simulink model "FinalProjectSimulinkModel_STAIRS"  (R2023b)
settings: Solver=VariableStepAuto  StartTime=0.0  StopTime=5  RelTol=1e-3
values from neighbouring files (symbols this model uses):
  dq_d_COM = [0.75; 0; 0; 0; 0; 0]    [FinalProject_init.m]
  dtMPC = 0.03    [FinalProject_init.m]
  firstStairDist = 0.26    [FinalProject_init.m]
  kd_swing = 10    [FinalProject_init.m]
  kp_swing = 300    [FinalProject_init.m]
  kStep = 0.001    [FinalProject_init.m]
  NMPC = 10    [FinalProject_init.m]
  offsets = [0;tSwing;tSwing;0]    [FinalProject_init.m]
  q_hip_roll_i = 0    [FinalProject_init.m]
  Qmpc = diag([100 100 50 1000 1000 500 4 4 4 1 1 1 0])    [FinalProject_init.m]
  Rmpc = 0.00001*eye(12)    [FinalProject_init.m]
  task = 6    [FinalProject_init.m]
  tCycle = 0.3    [FinalProject_init.m]
  tRamp = 0.5    [FinalProject_init.m]
  tSwing = tCycle/2    (= 0.15)    [FinalProject_init.m]
  x0_Trunk = [0;0;z_trunk_i-.15; 0;-0.271;0]    [FinalProject_init.m]
undefined symbols (not defined in the file or in its folder): X, Y, Z
libraries: sm_lib x208, nesl_utility x53
(part 5 of 5)

== system FinalProjectSimulinkModel_STAIRS/Rear Right Leg/Rear Right Thigh/RR_thigh ==
  Inertia : sm_lib/Body Elements/Inertia  InertiaType=Custom  Mass=1.013  MassUnits=kg  CenterOfMass=[0, 0, 0]  CenterOfMassUnits=m  MomentsOfInertia=[0.005529065, 0.005139339, 0.001367788]  MomentsOfInertiaUnits=kg*m^2  ProductsOfInertia=[-2.2448e-05, 0.000343869, -4.825e-06]  ProductsOfInertiaUnits=kg*m^2  GraphicType=None  MarkerShape=Inertia  MarkerSize=20  GraphicVisPropType=SimpleVisualProperties  GraphicDiffuseColor=[0.5 0.5 0.5]  GraphicSpecularColor=[0.5 0.5 0.5 1.0]  GraphicAmbientColor=[0.15 0.15 0.15 1.0]  GraphicEmissiveColor=[0.0 0.0 0.0 1.0]  GraphicShininess=75  GraphicOpacity=1.0
  InertiaOriginTransform : sm_lib/Frames and Transforms/Rigid Transform  TranslationMethod=Cartesian  TranslationStandardOffset=0  TranslationStandardOffsetUnits=m  TranslationStandardAxis=+Z  TranslationCartesianOffset=[-0.003237, 0.022327, -0.027326]  TranslationCartesianOffsetUnits=m  TranslationROffset=0  TranslationROffsetUnits=m  TranslationZOffset=0  TranslationZOffsetUnits=m  TranslationThetaOffset=0  TranslationThetaOffsetUnits=deg  RotationMethod=RotationSequence  RotationAngleUnits=deg  RotationStandardAxis=+Z  RotationAngle=0.0  RotationArbitraryAxis=[0 0 1]  FollAlignAxisA=+X  BaseAlignAxisA=+Y  FollAlignAxisB=+Y  BaseAlignAxisB=+Z  RotationSequenceAxes=BaseAxes  RotationSequence=XYZ  RotationSequenceAngles=[0, 0, 0]  RotationSequenceAnglesUnits=rad  RotationMatrix=[1 0 0; 0 1 0; 0 0 1]  Quaternion=[1 0 0 0]
  RR_calf_joint_AxisTransform : sm_lib/Frames and Transforms/Rigid Transform  TranslationMethod=Cartesian  TranslationStandardOffset=0  TranslationStandardOffsetUnits=m  TranslationStandardAxis=+Z  TranslationCartesianOffset=[0, 0, 0]  TranslationCartesianOffsetUnits=m  TranslationROffset=0  TranslationROffsetUnits=m  TranslationZOffset=0  TranslationZOffsetUnits=m  TranslationThetaOffset=0  TranslationThetaOffsetUnits=deg  RotationMethod=ArbitraryAxis  RotationAngleUnits=rad  RotationStandardAxis=+Z  RotationAngle=1.570796326794897  RotationArbitraryAxis=[-1, 0, 0]  FollAlignAxisA=+X  BaseAlignAxisA=+Y  FollAlignAxisB=+Y  BaseAlignAxisB=+Z  RotationSequenceAxes=FollowerAxes  RotationSequence=XYX  RotationSequenceAngles=[0 0 0]  RotationSequenceAnglesUnits=deg  RotationMatrix=[1 0 0; 0 1 0; 0 0 1]  Quaternion=[1 0 0 0]
  RR_calf_joint_OriginTransform : sm_lib/Frames and Transforms/Rigid Transform  TranslationMethod=Cartesian  TranslationStandardOffset=0  TranslationStandardOffsetUnits=m  TranslationStandardAxis=+Z  TranslationCartesianOffset=[0, 0, -0.2]  TranslationCartesianOffsetUnits=m  TranslationROffset=0  TranslationROffsetUnits=m  TranslationZOffset=0  TranslationZOffsetUnits=m  TranslationThetaOffset=0  TranslationThetaOffsetUnits=deg  RotationMethod=RotationSequence  RotationAngleUnits=deg  RotationStandardAxis=+Z  RotationAngle=0.0  RotationArbitraryAxis=[0 0 1]  FollAlignAxisA=+X  BaseAlignAxisA=+Y  FollAlignAxisB=+Y  BaseAlignAxisB=+Z  RotationSequenceAxes=BaseAxes  RotationSequence=XYZ  RotationSequenceAngles=[0, 0, 0]  RotationSequenceAnglesUnits=rad  RotationMatrix=[1 0 0; 0 1 0; 0 0 1]  Quaternion=[1 0 0 0]
  RR_thigh_joint_AxisInvTransform : sm_lib/Frames and Transforms/Rigid Transform  TranslationMethod=Cartesian  TranslationStandardOffset=0  TranslationStandardOffsetUnits=m  TranslationStandardAxis=+Z  TranslationCartesianOffset=[0, 0, 0]  TranslationCartesianOffsetUnits=m  TranslationROffset=0  TranslationROffsetUnits=m  TranslationZOffset=0  TranslationZOffsetUnits=m  TranslationThetaOffset=0  TranslationThetaOffsetUnits=deg  RotationMethod=ArbitraryAxis  RotationAngleUnits=rad  RotationStandardAxis=+Z  RotationAngle=1.570796326794897  RotationArbitraryAxis=[-1, 0, 0]  FollAlignAxisA=+X  BaseAlignAxisA=+Y  FollAlignAxisB=+Y  BaseAlignAxisB=+Z  RotationSequenceAxes=FollowerAxes  RotationSequence=XYX  RotationSequenceAngles=[0 0 0]  RotationSequenceAnglesUnits=deg  RotationMatrix=[1 0 0; 0 1 0; 0 0 1]  Quaternion=[1 0 0 0]
  ReferenceFrame : sm_lib/Frames and Transforms/Reference Frame
  Visual : sm_lib/Body Elements/File Solid  ExtGeomFileName=a1_description/meshes/thigh_mirror.stl  UnitType=Custom  ExtGeomFileUnits=m  StepReaderType=HEX  ExportConvexHullGeometry=off  InertiaType=Custom  Mass=0  MassUnits=kg  CenterOfMass=[0, 0, 0]  CenterOfMassUnits=m  MomentsOfInertia=[0, 0, 0]  MomentsOfInertiaUnits=kg*m^2  ProductsOfInertia=[0, 0, 0]  ProductsOfInertiaUnits=kg*m^2  BasedOnType=DensityFromFile  Density=1000  DensityUnits=kg/m^3  DoExposeReferenceFrame=on  SerializedFrames=<Frames/>  GraphicType=FromGeometry  MarkerShape=Sphere  MarkerSize=10  GraphicVisPropType=SimpleVisualProperties  GraphicDiffuseColor=[0.6 0.6 0.6]  GraphicSpecularColor=[0.5 0.5 0.5 1.0]  GraphicAmbientColor=[0.15 0.15 0.15 1.0]  GraphicEmissiveColor=[0.0 0.0 0.0 1.0]  GraphicShininess=75  GraphicOpacity=1
  VisualOriginTransform : sm_lib/Frames and Transforms/Rigid Transform  TranslationMethod=Cartesian  TranslationStandardOffset=0  TranslationStandardOffsetUnits=m  TranslationStandardAxis=+Z  TranslationCartesianOffset=[0, 0, 0]  TranslationCartesianOffsetUnits=m  TranslationROffset=0  TranslationROffsetUnits=m  TranslationZOffset=0  TranslationZOffsetUnits=m  TranslationThetaOffset=0  TranslationThetaOffsetUnits=deg  RotationMethod=RotationSequence  RotationAngleUnits=deg  RotationStandardAxis=+Z  RotationAngle=0.0  RotationArbitraryAxis=[0 0 1]  FollAlignAxisA=+X  BaseAlignAxisA=+Y  FollAlignAxisB=+Y  BaseAlignAxisB=+Z  RotationSequenceAxes=BaseAxes  RotationSequence=XYZ  RotationSequenceAngles=[0, 0, 0]  RotationSequenceAnglesUnits=rad  RotationMatrix=[1 0 0; 0 1 0; 0 0 1]  Quaternion=[1 0 0 0]
  F : PMIOPort  Side=Left
  F1 : PMIOPort  Port=2  Side=Right
  connections:
  Inertia/RConn1 -- InertiaOriginTransform/RConn1
  RR_calf_joint_AxisTransform/RConn1 -- F1/RConn1
  RR_calf_joint_AxisTransform/LConn1 -- RR_calf_joint_OriginTransform/RConn1
  RR_thigh_joint_AxisInvTransform/RConn1 -- F/RConn1
  RR_calf_joint_OriginTransform/LConn1 -- InertiaOriginTransform/LConn1 -- ReferenceFrame/RConn1 -- VisualOriginTransform/LConn1 -- RR_thigh_joint_AxisInvTransform/LConn1
  Visual/RConn1 -- VisualOriginTransform/RConn1

== system FinalProjectSimulinkModel_STAIRS/Rear Right Leg/Rear Right Calf and Foot/RR_calf ==
  Inertia : sm_lib/Body Elements/Inertia  InertiaType=Custom  Mass=0.166  MassUnits=kg  CenterOfMass=[0, 0, 0]  CenterOfMassUnits=m  MomentsOfInertia=[0.002997972, 0.003014022, 3.2426e-05]  MomentsOfInertiaUnits=kg*m^2  ProductsOfInertia=[0, -0.000141163, 0]  ProductsOfInertiaUnits=kg*m^2  GraphicType=None  MarkerShape=Inertia  MarkerSize=20  GraphicVisPropType=SimpleVisualProperties  GraphicDiffuseColor=[0.5 0.5 0.5]  GraphicSpecularColor=[0.5 0.5 0.5 1.0]  GraphicAmbientColor=[0.15 0.15 0.15 1.0]  GraphicEmissiveColor=[0.0 0.0 0.0 1.0]  GraphicShininess=75  GraphicOpacity=1.0
  InertiaOriginTransform : sm_lib/Frames and Transforms/Rigid Transform  TranslationMethod=Cartesian  TranslationStandardOffset=0  TranslationStandardOffsetUnits=m  TranslationStandardAxis=+Z  TranslationCartesianOffset=[0.006435, 0, -0.107388]  TranslationCartesianOffsetUnits=m  TranslationROffset=0  TranslationROffsetUnits=m  TranslationZOffset=0  TranslationZOffsetUnits=m  TranslationThetaOffset=0  TranslationThetaOffsetUnits=deg  RotationMethod=RotationSequence  RotationAngleUnits=deg  RotationStandardAxis=+Z  RotationAngle=0.0  RotationArbitraryAxis=[0 0 1]  FollAlignAxisA=+X  BaseAlignAxisA=+Y  FollAlignAxisB=+Y  BaseAlignAxisB=+Z  RotationSequenceAxes=BaseAxes  RotationSequence=XYZ  RotationSequenceAngles=[0, 0, 0]  RotationSequenceAnglesUnits=rad  RotationMatrix=[1 0 0; 0 1 0; 0 0 1]  Quaternion=[1 0 0 0]
  RR_calf_joint_AxisInvTransform : sm_lib/Frames and Transforms/Rigid Transform  TranslationMethod=Cartesian  TranslationStandardOffset=0  TranslationStandardOffsetUnits=m  TranslationStandardAxis=+Z  TranslationCartesianOffset=[0, 0, 0]  TranslationCartesianOffsetUnits=m  TranslationROffset=0  TranslationROffsetUnits=m  TranslationZOffset=0  TranslationZOffsetUnits=m  TranslationThetaOffset=0  TranslationThetaOffsetUnits=deg  RotationMethod=ArbitraryAxis  RotationAngleUnits=rad  RotationStandardAxis=+Z  RotationAngle=1.570796326794897  RotationArbitraryAxis=[-1, 0, 0]  FollAlignAxisA=+X  BaseAlignAxisA=+Y  FollAlignAxisB=+Y  BaseAlignAxisB=+Z  RotationSequenceAxes=FollowerAxes  RotationSequence=XYX  RotationSequenceAngles=[0 0 0]  RotationSequenceAnglesUnits=deg  RotationMatrix=[1 0 0; 0 1 0; 0 0 1]  Quaternion=[1 0 0 0]
  RR_foot_fixed_OriginTransform : sm_lib/Frames and Transforms/Rigid Transform  TranslationMethod=Cartesian  TranslationStandardOffset=0  TranslationStandardOffsetUnits=m  TranslationStandardAxis=+Z  TranslationCartesianOffset=[0, 0, -0.2]  TranslationCartesianOffsetUnits=m  TranslationROffset=0  TranslationROffsetUnits=m  TranslationZOffset=0  TranslationZOffsetUnits=m  TranslationThetaOffset=0  TranslationThetaOffsetUnits=deg  RotationMethod=RotationSequence  RotationAngleUnits=deg  RotationStandardAxis=+Z  RotationAngle=0.0  RotationArbitraryAxis=[0 0 1]  FollAlignAxisA=+X  BaseAlignAxisA=+Y  FollAlignAxisB=+Y  BaseAlignAxisB=+Z  RotationSequenceAxes=BaseAxes  RotationSequence=XYZ  RotationSequenceAngles=[0, 0, 0]  RotationSequenceAnglesUnits=rad  RotationMatrix=[1 0 0; 0 1 0; 0 0 1]  Quaternion=[1 0 0 0]
  ReferenceFrame : sm_lib/Frames and Transforms/Reference Frame
  Visual : sm_lib/Body Elements/File Solid  ExtGeomFileName=a1_description/meshes/calf.stl  UnitType=Custom  ExtGeomFileUnits=m  StepReaderType=HEX  ExportConvexHullGeometry=off  InertiaType=Custom  Mass=0  MassUnits=kg  CenterOfMass=[0, 0, 0]  CenterOfMassUnits=m  MomentsOfInertia=[0, 0, 0]  MomentsOfInertiaUnits=kg*m^2  ProductsOfInertia=[0, 0, 0]  ProductsOfInertiaUnits=kg*m^2  BasedOnType=DensityFromFile  Density=1000  DensityUnits=kg/m^3  DoExposeReferenceFrame=on  SerializedFrames=<Frames/>  GraphicType=FromGeometry  MarkerShape=Sphere  MarkerSize=10  GraphicVisPropType=SimpleVisualProperties  GraphicDiffuseColor=[0.2 0.2 0.2]  GraphicSpecularColor=[0.5 0.5 0.5 1.0]  GraphicAmbientColor=[0.15 0.15 0.15 1.0]  GraphicEmissiveColor=[0.0 0.0 0.0 1.0]  GraphicShininess=75  GraphicOpacity=1
  VisualOriginTransform : sm_lib/Frames and Transforms/Rigid Transform  TranslationMethod=Cartesian  TranslationStandardOffset=0  TranslationStandardOffsetUnits=m  TranslationStandardAxis=+Z  TranslationCartesianOffset=[0, 0, 0]  TranslationCartesianOffsetUnits=m  TranslationROffset=0  TranslationROffsetUnits=m  TranslationZOffset=0  TranslationZOffsetUnits=m  TranslationThetaOffset=0  TranslationThetaOffsetUnits=deg  RotationMethod=RotationSequence  RotationAngleUnits=deg  RotationStandardAxis=+Z  RotationAngle=0.0  RotationArbitraryAxis=[0 0 1]  FollAlignAxisA=+X  BaseAlignAxisA=+Y  FollAlignAxisB=+Y  BaseAlignAxisB=+Z  RotationSequenceAxes=BaseAxes  RotationSequence=XYZ  RotationSequenceAngles=[0, 0, 0]  RotationSequenceAnglesUnits=rad  RotationMatrix=[1 0 0; 0 1 0; 0 0 1]  Quaternion=[1 0 0 0]
  F : PMIOPort  Side=Left
  F1 : PMIOPort  Port=2  Side=Right
  connections:
  Inertia/RConn1 -- InertiaOriginTransform/RConn1
  RR_calf_joint_AxisInvTransform/RConn1 -- F/RConn1
  RR_foot_fixed_OriginTransform/RConn1 -- F1/RConn1
  RR_calf_joint_AxisInvTransform/LConn1 -- InertiaOriginTransform/LConn1 -- ReferenceFrame/RConn1 -- VisualOriginTransform/LConn1 -- RR_foot_fixed_OriginTransform/LConn1
  Visual/RConn1 -- VisualOriginTransform/RConn1

== system FinalProjectSimulinkModel_STAIRS/Rear Right Leg/Rear Right Calf and Foot/RR_foot ==
  Inertia : sm_lib/Body Elements/Inertia  InertiaType=Custom  Mass=0.06  MassUnits=kg  CenterOfMass=[0, 0, 0]  CenterOfMassUnits=m  MomentsOfInertia=[9.6e-06, 9.6e-06, 9.6e-06]  MomentsOfInertiaUnits=kg*m^2  ProductsOfInertia=[0, 0, 0]  ProductsOfInertiaUnits=kg*m^2  GraphicType=None  MarkerShape=Inertia  MarkerSize=20  GraphicVisPropType=SimpleVisualProperties  GraphicDiffuseColor=[0.5 0.5 0.5]  GraphicSpecularColor=[0.5 0.5 0.5 1.0]  GraphicAmbientColor=[0.15 0.15 0.15 1.0]  GraphicEmissiveColor=[0.0 0.0 0.0 1.0]  GraphicShininess=75  GraphicOpacity=1.0
  InertiaOriginTransform : sm_lib/Frames and Transforms/Rigid Transform  TranslationMethod=Cartesian  TranslationStandardOffset=0  TranslationStandardOffsetUnits=m  TranslationStandardAxis=+Z  TranslationCartesianOffset=[0, 0, 0]  TranslationCartesianOffsetUnits=m  TranslationROffset=0  TranslationROffsetUnits=m  TranslationZOffset=0  TranslationZOffsetUnits=m  TranslationThetaOffset=0  TranslationThetaOffsetUnits=deg  RotationMethod=RotationSequence  RotationAngleUnits=deg  RotationStandardAxis=+Z  RotationAngle=0.0  RotationArbitraryAxis=[0 0 1]  FollAlignAxisA=+X  BaseAlignAxisA=+Y  FollAlignAxisB=+Y  BaseAlignAxisB=+Z  RotationSequenceAxes=BaseAxes  RotationSequence=XYZ  RotationSequenceAngles=[0, 0, 0]  RotationSequenceAnglesUnits=rad  RotationMatrix=[1 0 0; 0 1 0; 0 0 1]  Quaternion=[1 0 0 0]
  ReferenceFrame : sm_lib/Frames and Transforms/Reference Frame
  Visual : sm_lib/Body Elements/Spherical Solid  GraphicAmbientColor=[0.15 0.15 0.15 1.0]  BasedOnType=Density  CenterOfMass=[0, 0, 0]  CenterOfMassUnits=m  GraphicDiffuseColor=[1, 0.423529411765, 0.0392156862745]  Density=1000  DensityUnits=kg/m^3  DoExposeReferenceFrame=on  GraphicEmissiveColor=[0.0 0.0 0.0 1.0]  ExportEntireGeometry=on  SerializedExposedGeometries=<exposedGeometries><exposedGeom><rawGeomId>entire</rawGeomId><exposedGeomId>G</exposedGeomId></exposedGeom></exposedGeometries>  SerializedFrames=<Frames/>  MarkerShape=Sphere  MarkerSize=10  GraphicType=FromGeometry  InertiaType=Custom  Mass=0  MassUnits=kg  MomentsOfInertia=[0, 0, 0]  MomentsOfInertiaUnits=kg*m^2  GraphicOpacity=1  ProductsOfInertia=[0, 0, 0]  ProductsOfInertiaUnits=kg*m^2  GraphicShininess=75  GraphicSpecularColor=[0.5 0.5 0.5 1.0]  SphereRadius=.02  SphereRadiusUnits=m  GraphicVisPropType=SimpleVisualProperties
  VisualOriginTransform : sm_lib/Frames and Transforms/Rigid Transform  TranslationMethod=Cartesian  TranslationStandardOffset=0  TranslationStandardOffsetUnits=m  TranslationStandardAxis=+Z  TranslationCartesianOffset=[0, 0, 0]  TranslationCartesianOffsetUnits=m  TranslationROffset=0  TranslationROffsetUnits=m  TranslationZOffset=0  TranslationZOffsetUnits=m  TranslationThetaOffset=0  TranslationThetaOffsetUnits=deg  RotationMethod=RotationSequence  RotationAngleUnits=deg  RotationStandardAxis=+Z  RotationAngle=0.0  RotationArbitraryAxis=[0 0 1]  FollAlignAxisA=+X  BaseAlignAxisA=+Y  FollAlignAxisB=+Y  BaseAlignAxisB=+Z  RotationSequenceAxes=BaseAxes  RotationSequence=XYZ  RotationSequenceAngles=[0, 0, 0]  RotationSequenceAnglesUnits=rad  RotationMatrix=[1 0 0; 0 1 0; 0 0 1]  Quaternion=[1 0 0 0]
  F : PMIOPort  Side=Left
  G : PMIOPort  Port=2  Side=Right
  Foot Frame : PMIOPort  Port=3  Side=Right
  connections:
  Inertia/RConn1 -- InertiaOriginTransform/RConn1
  ReferenceFrame/RConn1 -- InertiaOriginTransform/LConn1 -- VisualOriginTransform/LConn1 -- F/RConn1
  Visual/RConn1 -- Foot Frame/RConn1 -- VisualOriginTransform/RConn1
  G/RConn1 -- Visual/LConn1

== system FinalProjectSimulinkModel_STAIRS/Front Left Leg/Front Left Hip/Front Left Hip Fixed/FL_thigh_shoulder ==
  ReferenceFrame : sm_lib/Frames and Transforms/Reference Frame
  F : PMIOPort  Side=Left
  connections:
  ReferenceFrame/RConn1 -- F/RConn1

== system FinalProjectSimulinkModel_STAIRS/Front Right Leg/Front Right Hip/Front Right Hip Fixed/FR_thigh_shoulder ==
  ReferenceFrame : sm_lib/Frames and Transforms/Reference Frame
  F : PMIOPort  Side=Left
  connections:
  ReferenceFrame/RConn1 -- F/RConn1

== system FinalProjectSimulinkModel_STAIRS/Rear Left Leg/Rear Left Hip/Rear Left Hip Fixed/RL_thigh_shoulder ==
  ReferenceFrame : sm_lib/Frames and Transforms/Reference Frame
  F : PMIOPort  Side=Left
  connections:
  ReferenceFrame/RConn1 -- F/RConn1

== system FinalProjectSimulinkModel_STAIRS/Rear Right Leg/Rear Right Hip/Rear Right Hip Fixed/RR_thigh_shoulder ==
  ReferenceFrame : sm_lib/Frames and Transforms/Reference Frame
  F : PMIOPort  Side=Left
  connections:
  ReferenceFrame/RConn1 -- F/RConn1

== matlab function FinalProjectSimulinkModel_STAIRS/MATLAB Function ==
  data: Q input; R output
function R = Q2Rotm(Q)
    % Extract quaternion components
    q0 = Q(1);
    q1 = Q(2);
    q2 = Q(3);
    q3 = Q(4);
    
    % Compute rotation matrix elements
    R11 = q0^2 + q1^2 - q2^2 - q3^2;
    R12 = 2*(q1*q2 - q0*q3);
    R13 = 2*(q0*q2 + q1*q3);
    R21 = 2*(q1*q2 + q0*q3);
    R22 = q0^2 - q1^2 + q2^2 - q3^2;
    R23 = 2*(q2*q3 - q0*q1);
    R31 = 2*(q1*q3 - q0*q2);
    R32 = 2*(q0*q1 + q2*q3);
    R33 = q0^2 - q1^2 - q2^2 + q3^2;
    
    % Construct rotation matrix
    RMat = [R11, R12, R13;
         R21, R22, R23;
         R31, R32, R33];

    R = reshape(RMat,[9,1]);
end

== matlab function FinalProjectSimulinkModel_STAIRS/Control Block/forceToTorqueMapping ==
  data: qTrunk input size=[12, 1]; qJ input size=[12, 1]; T output size=[12, 1]; F_SRBD input size=[12, 1]; pf_d input size=[12, 1]; pfi input size=[12, 1]; vF_d input size=[12, 1]; vfi input size=[12, 1]; contact input size=[4, 1]; kp_swing parameter; kd_swing parameter
function T = forceToTorqueMapping(qTrunk, qJ, F_SRBD, pf_d, pfi, vF_d, vfi, contact, kp_swing, kd_swing)

%Extract variables from input for each leg to split out and calculate
%torques
R = reshape(qTrunk(4:end), [3,3]);

%Commanded Forces
fd1 = F_SRBD(1:3);
fd2 = F_SRBD(4:6);
fd3 = F_SRBD(7:9);
fd4 = F_SRBD(10:12);

%Joint Angles
q1 = qJ(1:3);
q2 = qJ(4:6);
q3 = qJ(7:9);
q4 = qJ(10:12);

%Foot Positions
pf_1 = pfi(1:3);
pf_2 = pfi(4:6);
pf_3 = pfi(7:9);
pf_4 = pfi(10:12);

%Desired Foot Positions
pf_d1 = pf_d(1:3);
pf_d2 = pf_d(4:6);
pf_d3 = pf_d(7:9);
pf_d4 = pf_d(10:12);

%Foot Velocities
vf_1 = vfi(1:3);
vf_2 = vfi(4:6);
vf_3 = vfi(7:9);
vf_4 = vfi(10:12);

%Desired Foot Velocities
vf_d1 = vF_d(1:3);
vf_d2 = vF_d(4:6);
vf_d3 = vF_d(7:9);
vf_d4 = vF_d(10:12);

%Contact Status
contact1 = contact(1);
contact2 = contact(2);
contact3 = contact(3);
contact4 = contact(4);

%Calculate Joint Torques for Each Leg
T1 = computeDesiredTorque(R, fd1, q1, pf_1, vf_1, 1, pf_d1, vf_d1, contact1, kp_swing, kd_swing);
T2 = computeDesiredTorque(R, fd2, q2, pf_2, vf_2, 2, pf_d2, vf_d2, contact2, kp_swing, kd_swing);
T3 = computeDesiredTorque(R, fd3, q3, pf_3, vf_3, 3, pf_d3, vf_d3, contact3, kp_swing, kd_swing);
T4 = computeDesiredTorque(R, fd4, q4, pf_4, vf_4, 4, pf_d4, vf_d4, contact4, kp_swing, kd_swing);

%Concatenate
T = [T1; T2; T3; T4];

end

function T=computeDesiredTorque(R,fd,q,pf,vf,leg,pfd,vfd,contact, kp_swing, kd_swing)
    l1=0.045; % hip length
    l2=0.2; % thigh length
    l3=0.2; % calf length
    
    if leg==1 || leg==3 % left leg has sideSign 1
        sideSign=1;
    else
        sideSign=-1; % right leg has sideSign -1
    end
    s1=sin(q(1)); % for hip joint
    s2=sin(q(2)); % for thigh joint
    s3=sin(q(3)); % for calf joint
    
    c1=cos(q(1)); % for hip joint
    c2=cos(q(2)); % for thigh joint
    c3=cos(q(3)); % for calf joint
    
    c23=c2*c3-s2*s3;
    s23=s2*c3+c2*s3;

    J = zeros(3);
    
    J(1,1)=0;
    J(2,1)=-sideSign*l1*s1+l2*c2*c1+l3*c23*c1;
    J(3,1)=sideSign*l1*c1+l2*c2*s1+l3*c23*s1;
    
    J(1,2)=-l3*c23-l2*c2;
    J(2,2)=-l2*s2*s1-l3*s23*s1;
    J(3,2)=l2*s2*c1+l3*s23*c1;
    
    J(1,3)=-l3*c23;
    J(2,3)=-l3*s23*s1;
    J(3,3)=l3*s23*c1;

    %Compute Torques resulting from GRFs from MPC (will be 0 for any legs
    %not current in stance phase
    R=reshape(R,[3,3]);
    Rt=transpose(R);
    JT= transpose(J);
    T=-JT*Rt*fd;

    % For legs currently in swing phase, use a PD controller to track the
    % desired foot position as determined by foot Trajectory function
    if contact == 0
        T= JT*Rt*(kp_swing*(pfd-pf)+kd_swing*(vfd-vf));
    end

end

== matlab function FinalProjectSimulinkModel_STAIRS/Control Block/footInterp ==
  data: t input; pf_dT input; vf_dT input; pf_dk output; vf_dk output; tInterp input
function [pf_dk, vf_dk] = footInterp(t, pf_dT, vf_dT, tInterp)

% Generate a desired foot position and velocity for *tk* from a full
% trajectory.
pf_dk = zeros(12,1);
vf_dk = zeros(12,1);

%Loop over each foot
for ii = 1:4
    %Loop over each dimension (x,y,z)
    for jj = 1:3
       %Interpolate current desired foot location and position for current
       %time
       pf_dk(3*(ii-1)+jj, 1) = interp1(tInterp(:,ii), pf_dT(:,3*(ii-1)+jj), t, "linear", pf_dT(end,3*(ii-1)+jj)); 
       vf_dk(3*(ii-1)+jj, 1) = interp1(tInterp(:,ii), vf_dT(:,3*(ii-1)+jj), t, "linear", vf_dT(end,3*(ii-1)+jj)); 
    end
end

== matlab function FinalProjectSimulinkModel_STAIRS/Control Block/Desired COM State ==
  data: t input; x0 input; dqTrunk_d input; xD output; dtMPC parameter; NMPC parameter; tRamp parameter; task parameter
function xD = genXd(t, x0, dqTrunk_d, dtMPC, NMPC, tRamp, task)

% Generate a desired COM Position for each of the MPC steps given an
% initial position of the COM and the Desired velocity 

xD = zeros(13, 10);
g = 9.81;

% Generate a vector of times at which the upcoming MPC run will make
% predicitons
tVec = linspace(t+dtMPC, t+NMPC*dtMPC,NMPC);

%Stair Height
maxStairHeight = 0.5;
%Crouch Down Slightly
restingRobotHeight = 0.25;

%Loop over each MPC timestep
for ii = 1:NMPC
    t_k = tVec(ii);
    %Generate desired q and dq
    qd_k = gen_qd_k(t_k, x0, dqTrunk_d, tRamp);
    dqd_k = gen_dqd_k(t_k, dqTrunk_d, tRamp);

    %If the robot has reached the top of the stairs, keep the height
    %constant
    if task == 6 && qd_k(3) > (restingRobotHeight + maxStairHeight)
        qd_k(3) = (restingRobotHeight + maxStairHeight);
        dqd_k(3) = 0;
    end
    %concatenate into desired MPC state (including g) for the timestep
    xD(:,ii) = [qd_k;dqd_k; g];
end

end

function qd_k = gen_qd_k(t,x0, dq_Trunk_d, tRamp)
    %Function calculated qd_k given the desired velocity

    %Assuming Linear Ramp Up to desired velocity (constant accel)
    a = dq_Trunk_d/tRamp; %Calculate Constant Accel of Ramp

    if t <= tRamp
        %If less than ramp up time, trajectory is parabolic
        qd_k = x0 + (0.5)*a*t^2;
    else
        %If time is greater than ramp up time, trajectory is linear, with
        %an offset determined by the ramp up time
        qd_k = x0 + (0.5)*a*tRamp^2 + dq_Trunk_d*(t-tRamp); 
    end
end

function dqd_k = gen_dqd_k(t, dq_Trunk_d, tRamp)
    a = dq_Trunk_d/tRamp; %Calculate Constant Accel of Ramp    
    if t <= tRamp
        %If time is less than ramp up time, velocity is linear
        dqd_k = a*t;
    else
        %If time is greater than ramp up time velocity is constant
        dqd_k = dq_Trunk_d;
    end
end

== matlab function FinalProjectSimulinkModel_STAIRS/Control Block/Gait ==
  data: mpcTable output; currentContact output; t input; tSwing input; tCycle input; offsets input; NMPC parameter; dtMPC parameter
function [mpcTable, currentContact] = gait(t, tSwing, tCycle, offsets, NMPC, dtMPC)
    %Calculate how long the feet are in contact with the ground
    tContact = tCycle-tSwing;

    %Initialize the gait table   
    mpcTable = zeros(NMPC*4,1);

    %Loop through each MPC timestep
    for i = 0:NMPC-1
        %Calculate the overall phase in the gait cycle
        phase = mod(t + (i*dtMPC), tCycle);

        %Offset by individual foot offsets to get the phase of each leg       
        progress = phase*ones(4,1) - offsets(:);
    
        %Loop Through Each Leg and determine its mode at the timestep
        for j = 1:4
            if progress(j) < 0
                progress(j) = progress(j) + tCycle;
            end
            if progress(j) < tContact
                mpcTable(i*4+j) = 1;
            else
                mpcTable(i*4+j) = 0;
            end    
        end
    end
    %Output the first 4 entries at the current contact state
    currentContact = mpcTable(1:4);
end

== matlab function FinalProjectSimulinkModel_STAIRS/Control Block/motorDyn ==
  data: T_FL output; T_FR output; T_RL output; T input; T_RR output
function [T_FL, T_FR, T_RL, T_RR] = motorDyn(T)
%Enforce torque limit of motors prior to passing the torques to the
%simulation
torqueLimit = 33.5; %Nm

for ii = 1:max(size(T))
    if T(ii) > torqueLimit
        T(ii) = torqueLimit;
    elseif T(ii) < -torqueLimit
        T(ii) = -torqueLimit;
    end
end

%Split out torques into each leg in order to pass to simulation
T_FL = T(1:3);
T_FR = T(4:6);
T_RL = T(7:9);
T_RR = T(10:12);

== matlab function FinalProjectSimulinkModel_STAIRS/Control Block/MPC Controller ==
  data: tSim input; qTrunk input; dqTrunk input; xTrunk_d input; pfs input; F output; gaitMap input; F_Prev input; iter_prev input; NMPC parameter; dtMPC parameter; iter output size=[1,1]; Qmpc parameter; Rmpc parameter; yawPrev input; yaw output; firstStairDist parameter
function [F, iter, yaw] = SRBD_MPC(tSim, qTrunk, dqTrunk, xTrunk_d, pfs, gaitMap, F_Prev, iter_prev, NMPC, dtMPC, Qmpc, Rmpc, yawPrev, firstStairDist)
%%
%Run quadprog outside of Simulink environment - tested faster than using
%"active-set" in our testing
coder.extrinsic('quadprog');
coder.extrinsic('optimoptions')
F = zeros(12,1);

if floor(tSim/dtMPC) ~= iter_prev
    iter = floor(tSim/dtMPC);
    %Global Parameters
    g = 9.81;
    
    % Extract State Variables
    r = qTrunk(1:3); R = qTrunk(4:end);
    v = dqTrunk(1:3); wb = dqTrunk(4:end);
    
    %Reshape R into Rotation Matrix and get Euler Angles
    RMat = reshape(R,[3,3]);
    eul = flip(rotm2eul(RMat))';
    
    %Ensure that euler angles increase or descrease continuously with no
    %skips to prevent MPC from freaking out
    yawUnwrap = unwrap([yawPrev, eul(3)]);
    eul(3) = yawUnwrap(2);
    yaw = eul(3);
    
    %Generate state vector for MPC (RotMat to Euler angles, add g)
    stateMPC = [r;eul;v;wb;g];
    
    %Robot Parameters (Mass and Inertia Matrix)
    m = 12;
    
    Ixb = 0.0168; Iyb = 0.0565; Izb = 0.064;
    Ib = diag([Ixb, Iyb, Izb]);
    
    %%
    %Project Feet Positions down to ground for prediction steps!
    zf1 = projToStair(pfs(1), firstStairDist);
    pF1 = [pfs(1:2); zf1];
    zf2 = projToStair(pfs(4), firstStairDist);
    pF2 = [pfs(4:5); zf2];
    zf3 = projToStair(pfs(7), firstStairDist);
    pF3 = [pfs(7:8); zf3];
    zf4 = projToStair(pfs(10), firstStairDist);
    pF4 = [pfs(10:11); zf4];
    
    pFs = [pF1, pF2, pF3, pF4];
    
    %Generate MPC Constraints
    fmin = 10;
    fmax = 500;
    mu = 0.5;
    
    %Aqp Matrix Generation
    AqpTemp = [-1 0 -mu; 1 0 -mu; 0 -1 -mu; 0 1 -mu; 0 0 1; 0 0 -1];
    Aqp = kron(eye(4), AqpTemp);
    AqpMPCTemp = kron(eye(NMPC),Aqp);
    AqpMPC = [zeros(24*NMPC, 13*NMPC), AqpMPCTemp];
    
    %bqp vector generation
    bqp = repmat([0;0;0;0;fmax;-fmin], 4,1);
    %bqp matrix is modified based on whether a foot is on the ground or not
    %(enforces feet being on the ground or in swing phase)
    bqpMPC = kron(gaitMap,bqp(1:6));
    
    %Calculate H from Cost Function Matrices
    HMPCTemp1 = kron(eye(NMPC),Qmpc);
    HMPCTemp2 = kron(eye(NMPC),Rmpc);
    HMPC = blkdiag(HMPCTemp1, HMPCTemp2);
    
    %Calculate fT using desired state (time varyuing)
    fT = zeros(1, 25*NMPC);
    for ii = 1:NMPC
        fT(ii*13-12:ii*13) = -1* xTrunk_d(:,ii)'*Qmpc;
    end
    fMPC = fT';
    
    NForces = 12;
    
    %Generate Equality (dynamic) constraints
    Aeq = genAeq([qTrunk;dqTrunk],pFs, NMPC, dtMPC, m, Ib, eul);
    Ampc = genA_MPC(eul, dtMPC);
    Beq = [Ampc*stateMPC; zeros(13*(NMPC-1),1)];
    
    %Provide Initial Guess
    guessX0 = [repmat(stateMPC, [NMPC, 1]); repmat(F_Prev, [NMPC, 1])];
    
    %Run Quadprog
    options = optimoptions('quadprog','Display','off','Algorithm','interior-point-convex');
    optOut = quadprog(HMPC, fMPC, AqpMPC, bqpMPC, Aeq, Beq, [], [], guessX0, options);
    
    F(:) = optOut(13*NMPC+1:13*NMPC+NForces);
else
    %Otherwise output the previous force 
    F(:) = F_Prev;
    iter = iter_prev;
    yaw = yawPrev;
end

end

%% Helper Functions

function Ampc = genA_MPC(eul, dtMPC)
    ATemp = zeros(13);
    ATemp(1:3, 7:9) = eye(3);
    pitch = eul(2);
    yaw = eul(3);

    % SRBD Dynamics without linearizing assumption
    w2eul = [cos(yaw)/cos(pitch), sin(yaw)/cos(pitch), 0;
            -sin(yaw), cos(yaw), 0;
            cos(yaw)*tan(pitch), sin(yaw)*tan(pitch), 1];
    ATemp(4:6, 10:12) = w2eul;
    ATemp(7:9, 13) = [0,0,-1];

    Ampc = eye(size(ATemp)) + dtMPC*ATemp;
end

function Bmpc = genB_MPC(state, pFs, dtMPC, m, Ib)

    % Extract State Variables
    r = state(1:3);
    R = state(4:12);

    pF1 = pFs(:,1);
    pF2 = pFs(:,2);
    pF3 = pFs(:,3);
    pF4 = pFs(:,4);

    %Reshape R into Rotation Matrix
    RMat = reshape(R,[3,3]);

    %Calculate Inertia Matrix in World Frame
    Iw = RMat*Ib*RMat';

    %Calcuate Foot Positions relative to COM
    rPF1 = pF1-r;
    rPF2 = pF2-r;
    rPF3 = pF3-r;
    rPF4 = pF4-r;

    %SRBD Dyanmics 
    Bmpc = dtMPC*[zeros([6,12]);
    (1/m)*repmat(eye(3),1,4);
    Iw\skewOp(rPF1), Iw\skewOp(rPF2), Iw\skewOp(rPF3), Iw\skewOp(rPF4);
    zeros(1,12)];
end

function Aeq = genAeq(state, pFs, NMPC, dtMPC, m, Ib, eul)
    %Calculate Ak and Bk matrices 
    Ampc = genA_MPC(eul, dtMPC);
    Bmpc = genB_MPC(state, pFs, dtMPC, m, Ib);

    %Concatenate into Aeq matrix
    Aeq = [eye(13*NMPC) + kron(diag(ones(1,NMPC-1),-1), -Ampc), kron(diag(ones(1,NMPC)), -Bmpc)];
end

function skewMat  = skewOp(vec)
    %Calculate Skew Symmetric Transform
    skewMat = [ 0 -vec(3) vec(2);
                vec(3) 0  -vec(1);
                -vec(2) vec(1) 0];
end

function zFoot = projToStair(xFoot, firstStairDist)
    %Project the z value of the foot down to the ground
    stairHeight = 0.1;
    stairLength = 0.2;
    stairLookup = zeros(6, 2);
    stairLookup(1,1) = -1000000000000;
    for ii = 1:5
        stairLookup(ii+1,:) = [firstStairDist + (ii-1)*stairLength, ii*stairHeight];
    end

    zFoot = interp1(stairLookup(:,1), stairLookup(:,2), xFoot,'previous', max(stairLookup(:,2)));
end

== matlab function FinalProjectSimulinkModel_STAIRS/Control Block/footPlacement ==
  data: qTrunk input; pf_d output; dqTrunk input; tSwing input; dqTrunk_d input; contactChange input; pf_d_Prev input; task input; kStep parameter; firstStairDist parameter
function pf_d = footPlacement (qTrunk, dqTrunk, tSwing, dqTrunk_d, contactChange, pf_d_Prev, task, kStep, firstStairDist)

% qTrunk is the position and rotation matrix of the trunk
% dqTrunk is the linear and angular velocity of the trunk
% tSwing is the amount of time between leg "liftoff" and leg contact (NOT
% THE SAME AS TCYCLE)
%dqTrunk_d is the desired linear and angular velocity of the trunk
%contact is a 4x1 boolean representing the which feet are currently on the
%ground and which are currently in the air (1 = on the ground, 0 is in the
%air

%Generate stair lookup table
stairHeight = 0.1;
stairLength = 0.2;
stairLookup = zeros(6, 2);
stairLookup(1,1) = -1000000000000;
for ii = 1:5
    stairLookup(ii+1,:) = [firstStairDist + (ii-1)*stairLength, ii*stairHeight];
end

%Extract poisition, orientation, velocity, and desired velocity from input
p = qTrunk(1:3);
R = reshape(qTrunk(4:end),[3,3]);
vCOM = dqTrunk(1:3);
vCOMd = dqTrunk_d(1:3);


%Hip Locations in Body Frame
a = 0.1805*2; b = 0.1308*2; c = 0;
h1b = [a/2; b/2; -c/2];
h2b = [a/2; -b/2; -c/2];
h3b = [-a/2; b/2; -c/2];
h4b = [-a/2; -b/2; -c/2];
hb = [h1b, h2b, h3b, h4b];

pf_d = zeros(12,1);
%Loop over each foot
for ii = 1:4
    %Only run this segment if leg goes from in-contact to swing phase
    if contactChange(ii) < 0
        %Find Hip Locations in World Frame
        pHip_i = R*hb(:,ii)+p;
        if task == 4 %spinning in place
            pf_d_i = pHip_i; %Only consider hip position
        elseif task == 5
            pf_d_i = pHip_i + (tSwing/2)*vCOM*1.25 + kStep*(vCOM-vCOMd); % add a slight factor to place the foot further in front.
        else
            pf_d_i = pHip_i + (tSwing/2)*vCOM + kStep*(vCOM-vCOMd); % For most tasks, default approach is suitable
        end

        %Check the stair "deadband" then project Feet to the current stair location
        if task == 6
            xFoot = deadbandCheck(pf_d_i(1), stairLookup);
            pf_d_i(1) = xFoot;
            zFoot = projToStair(pf_d_i(1), stairLookup);
        else
            zFoot = 0;
        end

        %Set the desired z location of the foot to 0
        pf_d(3*ii-2:3*ii) = [pf_d_i(1:2);zFoot];
    else
        %If foot has not left the ground or is still in the air, pass the
        %previous value of desired foot location
        pf_d(3*ii-2:3*ii) = pf_d_Prev(3*ii-2:3*ii);
    end
end

end

function zFoot = projToStair(xFoot, stairLookup)
    zFoot = interp1(stairLookup(:,1), stairLookup(:,2), xFoot,'previous', max(stairLookup(:,2)));
end

function xFoot = deadbandCheck(xFootIn, stairLookup)
    [~, nearestIdx] = min(abs(stairLookup(:,1)-xFootIn));
    nearestStairX = stairLookup(nearestIdx,1);

    distToStair = xFootIn - nearestStairX;

    lowerDeadband = .07;
    upperDeadband = .03;
    upperToLowerTransition = 0.005;

    if distToStair < upperToLowerTransition && distToStair >= -1*lowerDeadband
        xFoot = nearestStairX - lowerDeadband;
    elseif distToStair < upperDeadband && distToStair >= 0
        xFoot = nearestStairX + upperDeadband;
    else
        xFoot = xFootIn;
    end
end

== matlab function FinalProjectSimulinkModel_STAIRS/Control Block/footTrajectory ==
  data: pfd input; pfs input; tsim input; pf_dT output; vf_dT output; tSwing input; contactchange input; pf_dT_Prev input; vf_dT_Prev input; tInterp output; tInterp_Prev input
function [pf_dT, vf_dT, tInterp] = footTrajectory(pfd, pfs, tsim, tSwing, contactchange, pf_dT_Prev, vf_dT_Prev, tInterp_Prev)

%Last three inputs are trajectory arrays created in the previous step.

%numPoints control how fine you want to discretize the trajectory
%ie. it can be lowered if simulation is too slow
    numPoints = 100;
    dt= tSwing/numPoints;
    if dt == 0
        dt = 0.0000001;
    end

%pfd and Pfs is a 12x1 matrix
    %Initial Feet Positions
    Pfs1=pfs(1:3);
    Pfs2=pfs(4:6);
    Pfs3=pfs(7:9);
    Pfs4=pfs(10:12);
    
    %Desired Feet positions
    Pfd1=pfd(1:3);
    Pfd2=pfd(4:6);
    Pfd3=pfd(7:9);
    Pfd4=pfd(10:12);


%{   
    contactchange is a 4x1 matrix that informs whether each feet are leaving
the ground. Using it, generation of trajectory while the feet is
still on the ground or in the air was prevented by if statements.
%}
    contactchange1=contactchange(1);
    contactchange2=contactchange(2);
    contactchange3=contactchange(3);
    contactchange4=contactchange(4);

    if contactchange1 < 0
        %Finding desired foot trajectory of each feet
        P1 = generateSwingTrajectory(Pfs1,Pfd1,numPoints);
        %Finding desired foot velocity of each feet
        V1=zeros(numPoints,3);
        V1(1,:)=(P1(2,:)-P1(1,:))/(dt);
        V1(numPoints,:)=(P1(numPoints,:)-P1(numPoints-1,:))/(dt);
            for ii = 1:numPoints-2
                V1(ii+1,:) = (P1(ii+2,:)-P1(ii,:))/(2*dt);
            end
        tarray1=transpose(linspace(tsim,tsim+tSwing,numPoints));
    else
        P1 = pf_dT_Prev(:,1:3);
        V1 = vf_dT_Prev(:,1:3);
        tarray1=tInterp_Prev(:,1);
    end

    if contactchange2 < 0
        %Finding desired foot trajectory of each feet
        P2= generateSwingTrajectory(Pfs2,Pfd2,numPoints);
        %Finding desired foot velocity of each feet
        V2=zeros(numPoints,3);
        V2(1,:)=(P2(2,:)-P2(1,:))/(dt);
        V2(numPoints,:)=(P2(numPoints,:)-P2(numPoints-1,:))/(dt);
            for ii = 1:numPoints-2
                V2(ii+1,:) = (P2(ii+2,:)-P2(ii,:))/(2*dt);
            end
        tarray2=transpose(linspace(tsim,tsim+tSwing,numPoints));
    else
        P2 = pf_dT_Prev(:,4:6);
        V2 = vf_dT_Prev(:,4:6);
        tarray2=tInterp_Prev(:,2);
    end

    if contactchange3 < 0
        %Finding desired foot trajectory of each feet
        P3= generateSwingTrajectory(Pfs3,Pfd3,numPoints);
        %Finding desired foot velocity of each feet
        V3=zeros(numPoints,3);
        V3(1,:)=(P3(2,:)-P3(1,:))/(dt);
        V3(numPoints,:)=(P3(numPoints,:)-P3(numPoints-1,:))/(dt);
            for ii = 1:numPoints-2
                V3(ii+1,:) = (P3(ii+2,:)-P3(ii,:))/(2*dt);
            end
        tarray3=transpose(linspace(tsim,tsim+tSwing,numPoints));
    else
        P3 = pf_dT_Prev(:,7:9);
        V3 = vf_dT_Prev(:,7:9);
        tarray3=tInterp_Prev(:,3);
    end

    if contactchange4 < 0
        %Finding desired foot trajectory of each feet
        P4= generateSwingTrajectory(Pfs4,Pfd4,numPoints);
        %Finding desired foot velocity of each feet
        V4=zeros(numPoints,3);
        V4(1,:)=(P4(2,:)-P4(1,:))/(dt);
        V4(numPoints,:)=(P4(numPoints,:)-P4(numPoints-1,:))/(dt);
            for ii = 1:numPoints-2
                V4(ii+1,:) = (P4(ii+2,:)-P4(ii,:))/(2*dt);
            end
        tarray4=transpose(linspace(tsim,tsim+tSwing,numPoints));
    else
        P4 = pf_dT_Prev(:,10:12);
        V4 = vf_dT_Prev(:,10:12);
        tarray4=tInterp_Prev(:,4);
    end

% Generate a function of Time

    pf_dT = [P1 P2 P3 P4];
    vf_dT = [V1 V2 V3 V4];
    tInterp =[tarray1 tarray2 tarray3 tarray4];

end
    function trajectory = generateSwingTrajectory(initPosition,finalPosition,numpoints)
        % Generate a swing trajectory using the De Casteljau algorithm.
        %
        % Inputs:
        %   - controlPoints: Matrix of control points defining the trajectory.
        %   - numPoints: Number of points to interpolate along the trajectory.
        %
        % Output:
        %   - trajectory: Matrix of interpolated points representing the swing trajectory.
    
        % Check if the number of control points is sufficient for Bezier curve

        numPoints = numpoints;
        
        
        initPosition = initPosition';
        finalPosition = finalPosition';
        swingHeightFlat = 0.03;
        swingHeightStair = 0.13;

        if abs(initPosition(3) - finalPosition(3)) > 0.01
            c = swingHeightStair;
        else
            c = swingHeightFlat;
        end
        peakPosition = (finalPosition + initPosition) / 2 + [0,0,c];
   
        controlPoints = [initPosition;
                        initPosition + (peakPosition - initPosition)/2;
                        peakPosition;
                        peakPosition + (finalPosition - peakPosition)/2;
                        finalPosition]; 
       
    
        if size(controlPoints, 1) < 4
            error('Insufficient control points for Bezier curve');
        end
    
        % Interpolate points along the trajectory using De Casteljau algorithm
        t = linspace(0, 1, numPoints);
        trajectory = zeros(numPoints, size(controlPoints, 2));
    
        for i = 1:numPoints
            % Evaluate Bezier curve at parameter t using De Casteljau algorithm
            trajectory(i, :) = deCasteljau(controlPoints, t(i));
        end
    end
    
    function [point] = deCasteljau(controlPoints, t)
        % Recursive De Casteljau algorithm for evaluating Bezier curve.
        %
        % Inputs:
        %   - controlPoints: Matrix of control points defining the Bezier curve.
        %   - t: Parameter value between 0 and 1.
        %
        % Output:
        %   - point: Interpolated point on the Bezier curve.
    
        if size(controlPoints, 1) == 1
            point = controlPoints;
        else
            % Interpolate between adjacent control points
            nextControlPoints = zeros(size(controlPoints, 1) - 1, size(controlPoints, 2));
            for i = 1:size(controlPoints, 1) - 1
                nextControlPoints(i, :) = (1 - t) * controlPoints(i, :) + t * controlPoints(i + 1, :);
            end
            % Recursively call De Casteljau
            point = deCasteljau(nextControlPoints, t);
        end
    end
